simulink model "lowpass_PCS"  (R2021a)
settings: Solver=VariableStepAuto  StartTime=0.0  StopTime=etime  RelTol=1e-3
values from neighbouring files (symbols this model uses):
  dtload = 0.1    [initset_dataload.m]
libraries: eeGeneralControl x1
settings Model: Creator=PowerSystemLab  LastModifiedBy=PowerSystemLab

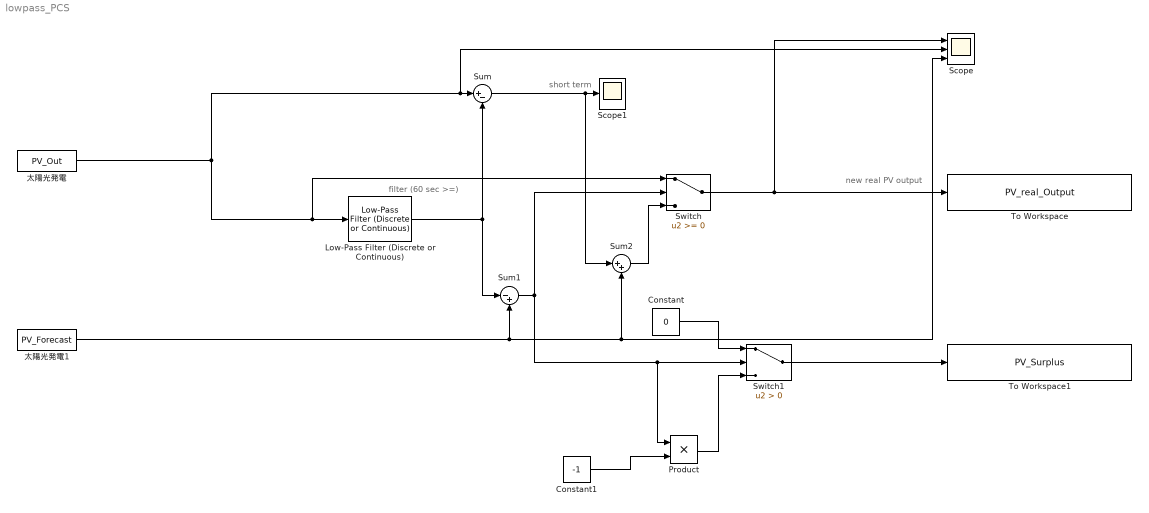
== system lowpass_PCS ==
  note: new real PV output
  note: short term
  note: filter (60 sec >=)
  Constant : Constant  Value=0
  Constant1 : Constant  Value=-1
  Low-Pass Filter (Discrete or Continuous) : eeGeneralControl/Low-Pass Filter (Discrete or Continuous)  K=1  T=1  B=inf  A=-inf  init_option=Inherited from block input  x0=0  Ts=-1
  Product : Product
  Scope : Scope  NumInputPorts=3
  Scope1 : Scope
  Sum : Sum  Inputs=|+-
  Sum1 : Sum  Inputs=|-+
  Sum2 : Sum  Inputs=|++
  Switch : Switch
  Switch1 : Switch  Criteria=u2 > Threshold
  To Workspace : ToWorkspace  VariableName=PV_real_Output  SampleTime=-1
      settings: Decimation=10
  To Workspace1 : ToWorkspace  VariableName=PV_Surplus  SampleTime=-1
      settings: Decimation=10
  太陽光発電 : FromFile  FileName=PV_Out  SampleTime=dtload
  太陽光発電1 : FromFile  FileName=PV_Forecast  SampleTime=dtload
  wires:
  太陽光発電1/1 -> Sum2/2, Scope/3, Sum1/2
  Low-Pass Filter (Discrete or Continuous)/1 -> Sum1/1, Sum/2
  Sum/1 -> Sum2/1, Scope1/1
  太陽光発電/1 -> Scope/2, Sum/1, Low-Pass Filter (Discrete or Continuous)/1, Switch/1
  Sum1/1 -> Product/1, Switch1/2, Switch/2
  Sum2/1 -> Switch/3
  Switch/1 -> Scope/1, To Workspace/1
  Constant/1 -> Switch1/1
  Constant1/1 -> Product/2
  Product/1 -> Switch1/3
  Switch1/1 -> To Workspace1/1
